simulink model "act2"  (R2021a)
settings: Solver=ode1  StartTime=0.0  StopTime=10.0  FixedStep=0.1  RelTol=1e-3
values from neighbouring files (symbols this model uses):
  a0 = 3    [exp1.m]
  a1 = 2    [exp1.m]    (also in main.m = 1)
  a2 = 1    [exp1.m]    (also in main.m = 2)
settings Model: Creator=zeta  LastModifiedBy=Agus

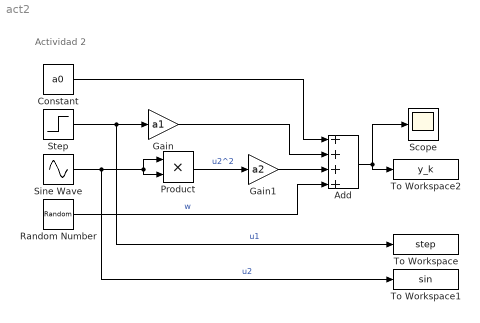
== system act2 ==
  note: Actividad 2
  Add : Sum  Inputs=++++
  Constant : Constant  Value=a0
  Gain : Gain  Gain=a1
  Gain1 : Gain  Gain=a2
  Product : Product
  Random Number : RandomNumber  Variance=0.1  Seed=round(rand()*100)  SampleTime=0.1
  Scope : Scope
  Sine Wave : Sin  Frequency=10  SampleTime=0
  Step : Step  SampleTime=0
  To Workspace : ToWorkspace  VariableName=step  SampleTime=0.5
  To Workspace1 : ToWorkspace  VariableName=sin  SampleTime=0.5
  To Workspace2 : ToWorkspace  VariableName=y_k  SampleTime=0.5
  wires:
  Add/1 -> To Workspace2/1, Scope/1
  Sine Wave/1 -> Product/2, Product/1, To Workspace1/1  "u2"
  Step/1 -> To Workspace/1, Gain/1  "u1"
  Random Number/1 -> Add/4  "w"
  Gain/1 -> Add/2
  Constant/1 -> Add/1
  Product/1 -> Gain1/1  "u2^2"
  Gain1/1 -> Add/3
